simulink model "MCP_phase3_redusedobsv"  (R2020a)
settings: Solver=VariableStepAuto  StartTime=0.0  StopTime=15.0  RelTol=1e-3
settings Model: Creator=rafiee  LastModifiedBy=Lenovo
settings DataIOCC: ReturnWorkspaceOutputs=off
settings DebuggingCC: ArithmeticOperatorsInVariantConditions=warning
settings SFSimCC: SimUseLocalCustomCode=off  CustomCodeUndefinedFunction=UseInterfaceOnly
settings RTWCC: RTWUseLocalCustomCode=off
settings CodeAppCC: StateflowObjectComments=on

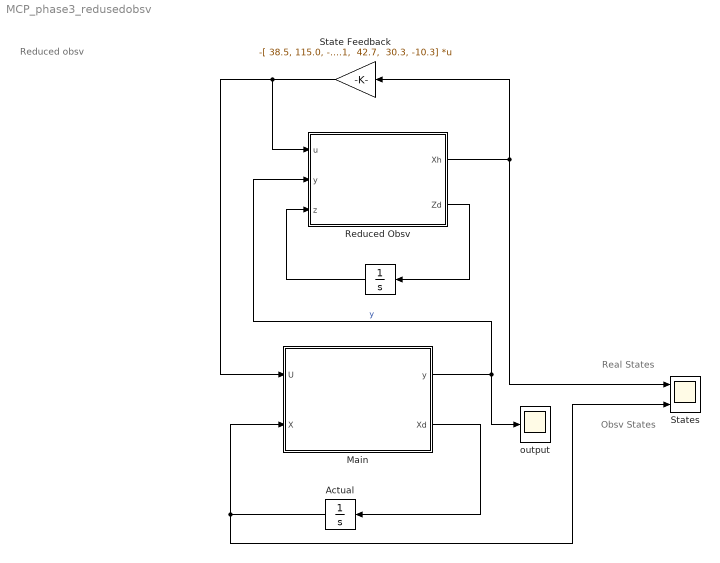
== system MCP_phase3_redusedobsv ==
  note: Real States
  note: Obsv States
  note: Reduced obsv
  " " : Integrator  InitialCondition=[0;0]
  Actual : Integrator  InitialCondition=[0.1;1;0.5;-1]
  Main : MATLAB Function  TreatAsAtomicUnit=on
  Reduced Obsv : MATLAB Function  TreatAsAtomicUnit=on
  State Feedback : Gain  Gain="-[ 38.5, 115.0, -55.3,  54.2; 38.1,  42.7,  30.3, -10.3]"  Multiplication=Matrix(K*u)
  States : Scope  NumInputPorts=2
  "output " : Scope
  wires:
  Main/1(y) -> "output "/1, Reduced Obsv/2(y)  "y"
  Reduced Obsv/1(Xh) -> States/1, State Feedback/1
  Main/2(Xd) -> Actual/1
  Reduced Obsv/2(Zd) -> " "/1
  State Feedback/1 -> Reduced Obsv/1(u), Main/1(U)
  " "/1 -> Reduced Obsv/3(z)
  Actual/1 -> Main/2(X), States/2

== matlab function MCP_phase3_redusedobsv/Main ==
  data: y output; U input size=[2,1]; Xd output size=[4,1]; X input size=[4,1]
function [y, Xd]  = linear_plant(U, X)

A = [ -0.0189,       0,  0.029,       0;
       0, -0.0191,      0,  0.0349;
       0,       0, -0.029,       0;
       0,       0,      0, -0.0349];
   
B =[ 0.00306,      0;
       0, 0.0035;
       0, 0.0065;
 0.00714,      0];


 C = [ 1.0,   0, 0, 0;
   0, 1.0, 0, 0];

Xd = A*X + B*U; 
y = C*X

== matlab function MCP_phase3_redusedobsv/Reduced Obsv ==
  data: Xh output; u input; Zd output; y input; z input
function [Xh, Zd]= Obsv_R(u , y, z)
% System main Matrices
B = [ 0.00306,      0;
       0, 0.0035;
       0, 0.0065;
 0.00714,      0];


 C = [ 1.0,   0, 0, 0;
   0, 1.0, 0, 0];

% Observer Matrices
F = [ -0.4,     0;
    0, -0.45];

T = [ 2.62,     0, -0.205,     0;
    0, -2.32,      0, 0.195];


L = [ 1.0,    0;
   0, -1.0];

Zd = F*z + T*B*u + L*y;
Xh = ([C;T]^-1)*[y;z];
end
